simulink model "Jacobianpartb"  (R2020b)
settings: Solver=VariableStepAuto  StartTime=0.0  StopTime=10.0  RelTol=1e-3
values from neighbouring files (symbols this model uses):
  l1 = 1    [run_sim_asn5q1.m]    (also in run_sim_asn5q1c.m)
  l2 = 1    [run_sim_asn5q1.m]    (also in run_sim_asn5q1c.m)
settings Model: Creator=huber  LastModifiedBy=huber

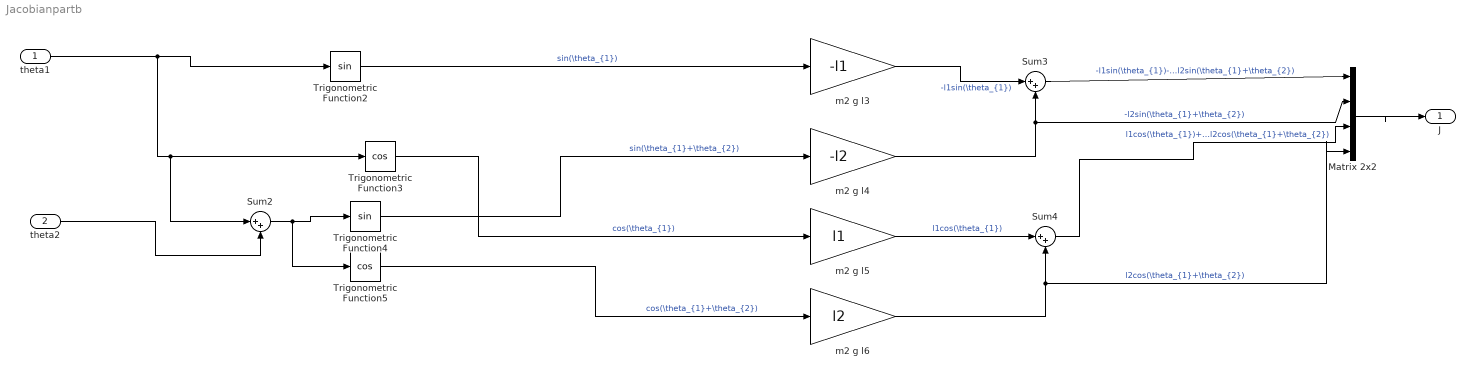
== system Jacobianpartb ==
  theta1 : Inport
  theta2 : Inport  Port=2
  Matrix 2x2 : Concatenate  NumInputs=4  Mode=Multidimensional array  ConcatenateDimension=2
  Sum2 : Sum  Inputs=|++
  Sum3 : Sum  Inputs=|++
  Sum4 : Sum  Inputs=|++
  Trigonometric Function2 : Trigonometry
  Trigonometric Function3 : Trigonometry  Operator=cos
  Trigonometric Function4 : Trigonometry
  Trigonometric Function5 : Trigonometry  Operator=cos
  m2 g l3 : Gain  Gain=-l1
  m2 g l4 : Gain  Gain=-l2
  m2 g l5 : Gain  Gain=l1
  m2 g l6 : Gain  Gain=l2
  J : Outport
  wires:
  m2 g l5/1 -> Sum4/1  "l1cos(\\theta_{1})"
  m2 g l6/1 -> Matrix 2x2/4, Sum4/2  "l2cos(\\theta_{1}+\\theta_{2})"
  Sum3/1 -> Matrix 2x2/1  "-l1sin(\\theta_{1})-l2sin(\\theta_{1}+\\theta_{2})"
  m2 g l3/1 -> Sum3/1  "-l1sin(\\theta_{1})"
  Trigonometric Function4/1 -> m2 g l4/1  "sin(\\theta_{1}+\\theta_{2})"
  Sum2/1 -> Trigonometric Function5/1, Trigonometric Function4/1
  theta2/1 -> Sum2/2
  Trigonometric Function2/1 -> m2 g l3/1  "sin(\\theta_{1})"
  theta1/1 -> Sum2/1, Trigonometric Function3/1, Trigonometric Function2/1
  m2 g l4/1 -> Sum3/2, Matrix 2x2/2  "-l2sin(\\theta_{1}+\\theta_{2})"
  Trigonometric Function5/1 -> m2 g l6/1  "cos(\\theta_{1}+\\theta_{2})"
  Trigonometric Function3/1 -> m2 g l5/1  "cos(\\theta_{1})"
  Sum4/1 -> Matrix 2x2/3  "l1cos(\\theta_{1})+l2cos(\\theta_{1}+\\theta_{2})"
  Matrix 2x2/1 -> J/1
